simulink model "MotorSpeedFirst"  (R2016a)
settings: Solver=FixedStepAuto  SolverMode=SingleTasking  StartTime=0.0  StopTime=10  FixedStep=0.001  RelTol=1e-3
libraries: arduino_io_lib x4
settings Model: ExtModeTrigDuration=2  Creator=gcampa  LastModifiedBy=syf
settings DataIOCC: LimitDataPoints=on  SaveFormat=Array  SignalLoggingSaveFormat=ModelDataLogs
settings OptimizationCC: OptimizeModelRefInitCode=on  LifeSpan=1  MaxStackSize=64
settings DebuggingCC: UnderspecifiedInitializationDetection=Classic  MergeDetectMultiDrivingBlocksExec=none  MultiTaskDSMMsg=warning  MultiTaskCondExecSysMsg=none
settings HardwareCC: ProdBitPerInt=16  ProdBitPerPointer=16  ProdLargestAtomicFloat=None  ProdWordSize=8  ProdHWDeviceType=Atmel->AVR
settings ModelReferenceCC: PropagateSignalLabelsOutOfModel=off
settings RTWCC: SystemTargetFile=ert.tlc  HardwareBoard=Arduino Uno  TemplateMakefile=ert_default_tmf  GenerateReport=on  RTWVerbose=off  Toolchain=Arduino AVR v1.6.1  BuildConfiguration=Faster Runs  IncludeHyperlinkInReport=on  LaunchReport=on  GenerateTraceInfo=on  GenerateTraceReport=on  GenerateTraceReportSl=on  GenerateTraceReportSf=on  GenerateTraceReportEml=on
settings CodeAppCC: ForceParamTrailComments=on  IgnoreCustomStorageClasses=off  OperatorAnnotations=on  SimulinkDataObjDesc=on  SFDataObjDesc=on  MATLABFcnDesc=on  InsertBlockDesc=on  MATLABSourceComments=on
settings ERTTargetCC: SupportContinuousTime=on  SupportVariableSizeSignals=on
settings ConfigComp: CovModelRefEnable=Off

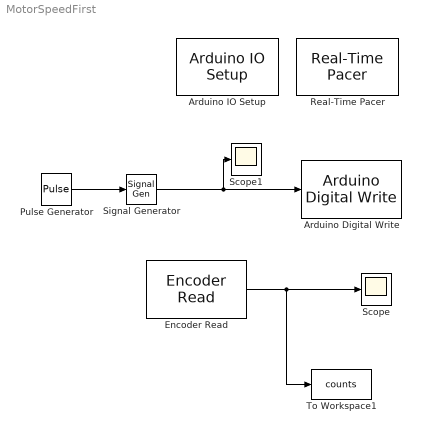
== system MotorSpeedFirst ==
  Arduino Digital Write : arduino_io_lib/Arduino Digital Write  arduinoVar=Temporary arduino variable: Arduino1  arduinoPin=5  T=-1
  Arduino IO Setup : arduino_io_lib/Arduino IO Setup  Priority=3  arduinoVar=Temporary arduino variable: Arduino1  workspaceVarName=b  comPort=COM4
  Encoder Read : arduino_io_lib/Encoder Read  arduinoVar=Temporary arduino variable: Arduino1  encNum=1  pinA=2  pinB=3  DbDl=0  T=0.01
  Pulse Generator : DiscretePulseGenerator  Period=10  PulseWidth=5  SampleTime=0.01
  Real-Time Pacer : arduino_io_lib/Real-Time Pacer  simTimePerRealTime=1
  Scope : Scope
  Scope1 : Scope
  Signal Generator : SignalGenerator  WaveForm=square  TimeSource=Use external signal  Frequency=10000  Units=rad/sec
  To Workspace1 : ToWorkspace  VariableName=counts  SaveFormat=Timeseries  SampleTime=-1
  wires:
  Signal Generator/1 -> Scope1/1, Arduino Digital Write/1
  Encoder Read/1 -> To Workspace1/1, Scope/1
  Pulse Generator/1 -> Signal Generator/1
